simulink library "INT_Fan_DD"  (R2016b)
settings: Solver=VariableStepAuto  StartTime=0.0  StopTime=10.0  RelTol=1e-3
settings Model: Creator=xinchangran  LastModifiedBy=xinchangran

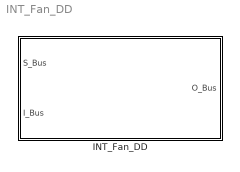
== system INT_Fan_DD ==
  INT_Fan_DD : Subsystem

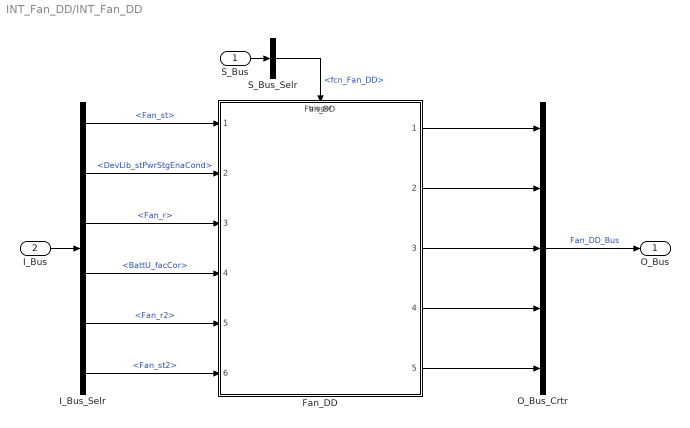
== system INT_Fan_DD/INT_Fan_DD ==
  S_Bus : Inport
  I_Bus : Inport  Port=2
  Fan_DD : ModelReference  ModelNameDialog=Fan_DD  SimulationMode=Normal  ModelReferenceVersion=1.95  TriggerPortName=function  TriggerPortTriggerType=function-call  TriggerPortStatesWhenEnabling=held
  I_Bus_Selr : BusSelector  OutputSignals=Fan_st,DevLib_stPwrStgEnaCond,Fan_r,BattU_facCor,Fan_r2,Fan_st2
  O_Bus_Crtr : BusCreator  Inputs=5
  S_Bus_Selr : BusSelector  OutputSignals=fcn_Fan_DD
  O_Bus : Outport
  wires:
  S_Bus_Selr/1 -> Fan_DD/Trigger  "<fcn_Fan_DD>"
  S_Bus/1 -> S_Bus_Selr/1
  I_Bus/1 -> I_Bus_Selr/1
  I_Bus_Selr/1 -> Fan_DD/1  "<Fan_st>"
  I_Bus_Selr/2 -> Fan_DD/2  "<DevLib_stPwrStgEnaCond>"
  I_Bus_Selr/3 -> Fan_DD/3  "<Fan_r>"
  I_Bus_Selr/4 -> Fan_DD/4  "<BattU_facCor>"
  I_Bus_Selr/5 -> Fan_DD/5  "<Fan_r2>"
  I_Bus_Selr/6 -> Fan_DD/6  "<Fan_st2>"
  O_Bus_Crtr/1 -> O_Bus/1  "Fan_DD_Bus"
  Fan_DD/1 -> O_Bus_Crtr/1
  Fan_DD/2 -> O_Bus_Crtr/2
  Fan_DD/3 -> O_Bus_Crtr/3
  Fan_DD/4 -> O_Bus_Crtr/4
  Fan_DD/5 -> O_Bus_Crtr/5
